simulink library "uDAQ28LT_lib"  (R2019b)
settings: Solver=VariableStepAuto  StartTime=0.0  StopTime=10.0  RelTol=1e-3
settings Model: Creator=dp  LastModifiedBy=dp

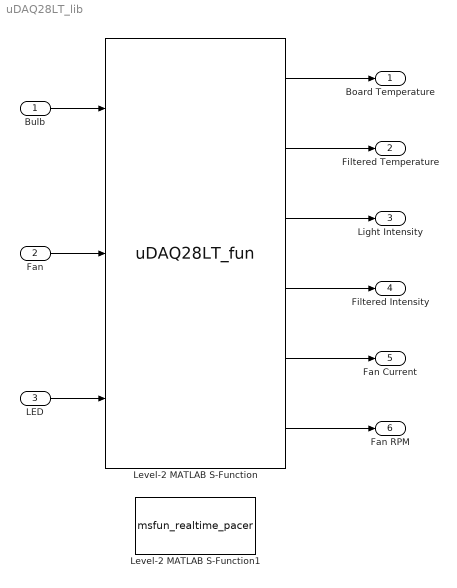
== system uDAQ28LT_lib ==
  Bulb : Inport
  Fan : Inport  Port=2
  LED : Inport  Port=3
  Level-2 MATLAB S-Function : M-S-Function  FunctionName=uDAQ28LT_fun  Parameters=com,baud,Ts  mask(uDAQ28LT Thermal plant Block){com='', baud=256000, Ts=0}
      mask prompts: com "COM port:"; baud "Baud rate:"; Ts "Sample period:"
      mask help: Simulink library for the uDAQ28/LT Thermal Plant.
      mask Display:
      | disp('uDAQ28/LT Thermal Plant')
      | 
      | port_label('input',1,'bulb')
      | port_label('input',2,'fan')
      | port_label('input',3,'led')
      | 
      | port_label('output',1,'temp')
      | port_label('output',2,'ftemp')
      | port_label('output',3,'intens')
      | port_label('output',4,'fintens')
      | port_label('output',5,'fanamp')
      | port_label('output',6,'fanrpm')
  Level-2 MATLAB S-Function1 : M-S-Function  FunctionName=msfun_realtime_pacer  Parameters=1  mask(RealTime_Pacer){simTimePerRealTime=1}
      mask prompts: simTimePerRealTime "Speedup (Simulation Time / Real Time):"
      mask help:
      | Slow down a simulation to track real (i.e., wall clock) elapsed time.
      |
      | "Speedup" specifies the ratio between simulation time and real time
      |  Speedup = N => N sec. of simulation time per sec. of real time
      |  Speedup can be fractional (e.g., 0.5, 1.3).
      |  Speedup = inf => allow simulation to run at full speed
      |
      | Click on the Help button for details.
      mask Display: disp('Real-Time Pacer')
  Board Temperature : Outport
  Filtered Temperature : Outport  Tag=Filtered Temperature  Port=2
  Light Intensity : Outport  Port=3
  Filtered Intensity : Outport  Port=4
  Fan Current : Outport  Port=5
  Fan RPM : Outport  Port=6
  wires:
  Level-2 MATLAB S-Function/2 -> Filtered Temperature/1
  Level-2 MATLAB S-Function/1 -> Board Temperature/1
  Level-2 MATLAB S-Function/3 -> Light Intensity/1
  Level-2 MATLAB S-Function/4 -> Filtered Intensity/1
  Level-2 MATLAB S-Function/5 -> Fan Current/1
  Level-2 MATLAB S-Function/6 -> Fan RPM/1
  Bulb/1 -> Level-2 MATLAB S-Function/1
  Fan/1 -> Level-2 MATLAB S-Function/2
  LED/1 -> Level-2 MATLAB S-Function/3
